simulink model "ResidentialBuildingTESandPVcell"  (R2023b)
settings: Solver=VariableStepAuto  StartTime=0.0  StopTime=3600*24  FixedStep=20  RelTol=1e-3  AbsTol=1e-3
PreLoadFcn:
  | setSystemParams
undefined symbols (not defined in the file): env, hours, htCondDuct, pumps, PVpanel, resUnitParams, tank, wCondDuct
libraries: fl_lib x137, nesl_utility x18, SimscapeFluids_lib x7, simulink x2, ee_lib x2, slpidlib x1
(part 1 of 3)
CloseFcn:
  | clear logsout_ResidentialBuildingTESandPVcell
  | 
  | clear PVpanel heatEx tank pumps TES env resUnitParams simTinit
Description:
  | PV charged sand battery for residential heating
settings Model: Creator=The MathWorks, Inc.  LastModifiedBy=shachind
settings SolverCC: AutoScaleAbsTol=off  MaxConsecutiveMinStep=5  ZeroCrossAlgorithm=Adaptive  AlgebraicLoopSolver=TrustRegion  MaxZcPerStep=1
settings DataIOCC: MaxDataPoints=10000  SaveOutput=off  DSMLogging=off  SaveTime=off  ReturnWorkspaceOutputs=off  SignalLoggingName=logsout_ResidentialBuildingTESandPVcell
settings OptimizationCC: ReuseModelBlockBuffer=off
settings DebuggingCC: ReadBeforeWriteMsg=DisableAll  WriteAfterWriteMsg=DisableAll  WriteAfterReadMsg=DisableAll  IgnoredZcDiagnostic=none  MultiTaskDSMMsg=none  UnconnectedInputMsg=warning  UnconnectedOutputMsg=warning  UnconnectedLineMsg=warning  ArithmeticOperatorsInVariantConditions=warning
settings ModelReferenceCC: UpdateModelReferenceTargets=IfOutOfDate  EnableRefExpFcnMdlSchedulingChecks=on
settings SFSimCC: SFSimEcho=off
settings RTWCC: DLArmComputeVersion=19.05
settings SimscapeCC: SimscapeLogType=all  SimscapeLogSimulationStatistics=on  SimscapeLogName=simlogResidentialBuildingTESandPVcell  SimscapeLogDecimation=10  SimscapeLogLimitData=off  SimscapeLogDataHistory=130000

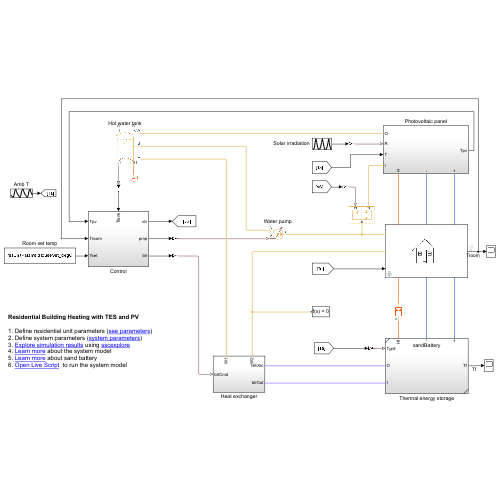
[thumbnail: Simulink's stored preview of the top-level diagram]
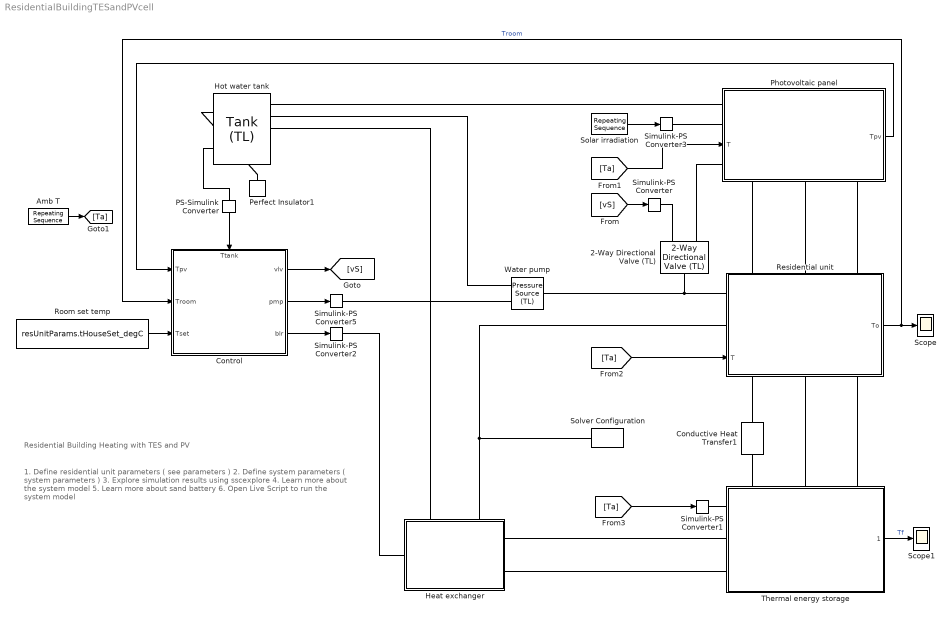
== system ResidentialBuildingTESandPVcell ==
  note: Residential Building Heating with TES and PV
  note: 1. Define residential unit parameters ( see parameters )
      | 2. Define system parameters ( system parameters )
      | 3. Explore simulation results using sscexplore
      | 4. Learn more about the system model
      | 5. Learn more about sand battery
      | 6. Open Live Script to run the system model
  " Water pump" : fl_lib/Thermal Liquid/Sources/Pressure Source (TL)  source_type=foundation.enum.constant_controlled.controlled  pressure_differential=0 MPa  power_spec=foundation.enum.power_spec.isentropic  area=0.01 m^2
      settings: InternalSimscapePortConfiguration="{\"Bottom\":[],\"Left\":[{\"id\":\"A\",\"label\":\"A\",\"type\":\"foundation.thermal_liquid.thermal_liquid\"},{\"id\":\"P\",\"label\":\"P\",\"type\":\"input\"}],\"Right\":[{\"id\":\"B\",\"label\":\"B\",\"type\":\"foundation.thermal_liquid.thermal_liquid\"}],\"Top\":[]}"
  2-Way Directional Valve (TL) : SimscapeFluids_lib/Thermal Liquid/Valves & Orifices/Directional Control Valves/2-Way Directional Valve (TL)  valve_spec=fluids.thermal_liquid.valves.directional_control_valves.enum.ValveSpec.Linear  S_max=5e-2 m  del_S_max=1e-1 m  area_max=2.5e-4 m^2  area_leak=1e-5 m^2  del_S_TLU=[0, .002, .004, .007, .017] m  valve_area_TLU=[1e-09, 2.0352e-07, 4.0736e-05, .00011438, .00034356] m^2  del_S_flow_TLU=[0, .002, .004, .007, .017] m  p_diff_TLU=[.3, .5, .7] MPa  vol_flow_TLU=1e-3 * [1.7e-05, 2e-05, 2.6e-05; .0035, .0045, .0053; .7, .9, 1.06; 1.96, 2.5, 3; 6, 7.7, 9.13] m^3/s  mdot_TLU=[1.7e-05, 2e-05, 2.6e-05; .0035, .0045, .0053; .7, .9, 1.06; 1.96, 2.5, 3; 6, 7.7, 9.13] kg/s  T_ref_in=293.15 K  p_ref_in=0.101325 MPa  Cd=0.7  Re_c=12  smoothing_factor=0.02  pressure_recovery=simscape.enum.onoff.off  area=0.01 m^2
      settings: InternalSimscapePortConfiguration="{\"Bottom\":[],\"Left\":[{\"id\":\"A\",\"label\":\"A\",\"type\":\"foundation.thermal_liquid.thermal_liquid\"}],\"Right\":[{\"id\":\"S\",\"label\":\"S\",\"type\":\"input\"},{\"id\":\"B\",\"label\":\"B\",\"type\":\"foundation.thermal_liquid.thermal_liquid\"}],\"Top\":[]}"
  Amb T : simulink/Sources/Repeating Sequence  rep_seq_t=3600*hours(env.hrs)  rep_seq_y=env.Temp_degC
  Conductive Heat Transfer1 : fl_lib/Thermal/Thermal Elements/Conductive Heat Transfer  thermal_type=foundation.enum.ConstantVariableTabulated.Constant  wall_geometry=foundation.enum.ConductionWallGeometry.Planar  area=TES.pitA m^2  thickness=0.5 m  d_in=0.05 m  d_out=0.1 m  L=1 m  th_cond_min=10 W/(K*m)  th_cond=3.5 W/(K*m)  th_cond_TLU=[413, 401, 392, 383, 371, 357, 342] W/(K*m)  temp_TLU=[200, 273, 400, 600, 800, 1000, 1200] K  T_specify=off  T_priority=None  T=0 K  T_nominal_specify=off  T_nominal_unit=K  T_nominal_value=1  Q_specify=off  Q_priority=None  Q=0 W  Q_nominal_specify=off  Q_nominal_unit=W  Q_nominal_value=1
  Control : Subsystem
      settings: PortSchema="{\"entries\":[{\"content\":{\"sides\":[{\"content\":{\"connectorIds\":[\"In1\",\"In2\",\"In3\"]},\"type\":\"ConnectorPlacement.EquallySpacedRectSide\",\"uuid\":\"94b2e64d-5198-497a-a3ac-7835c1f17d91\"},{\"content\":{\"connectorIds\":[\"Out1\",\"Out2\",\"Out3\"],\"side\":\"RIGHT\"},\"type\":\"ConnectorPlacement.EquallySpacedRectSide\",\"uuid\":\"aae50087-a35d-4e17-a15b-734053a702a5\"},{\"content\":{\"connectorIds\":[\"In4\"],\"side\":\"TOP\"},\"type\":\"ConnectorPlacement.EquallySpacedRectSide\",\"uuid\":\"cdfabfa3-3647-473e-9efb-0f4c40dd4bf4\"}]},\"type\":\"ConnectorPlacement.EquallySpacedConnector\",\"uuid\":\"f6b74bbd-681f-4865-9cfd-f9bd6391df02\"}],\"packageUris\":[\"http://schema.mathworks.com/mf0/Connector/R2020b\"],\"version\":\"1.0\"}"
  Heat exchanger : Subsystem
      settings: PortSchema="{\"entries\":[{\"content\":{\"sides\":[{\"content\":{\"connectorIds\":[\"LConn1\"]},\"type\":\"ConnectorPlacement.EquallySpacedRectSide\",\"uuid\":\"01ab44eb-c12d-4ed2-868c-d9720820a3c1\"},{\"content\":{\"connectorIds\":[\"RConn1\",\"RConn2\"],\"side\":\"RIGHT\"},\"type\":\"ConnectorPlacement.EquallySpacedRectSide\",\"uuid\":\"0fee6253-0b63-4bf2-bc48-ef503382f712\"},{\"content\":{\"connectorIds\":[\"LConn2\",\"LConn3\"],\"side\":\"TOP\"},\"type\":\"ConnectorPlacement.EquallySpacedRectSide\",\"uuid\":\"0da63f1e-723a-4e43-a092-4a52b54a8044\"}]},\"type\":\"ConnectorPlacement.EquallySpacedConnector\",\"uuid\":\"e3ac5915-ab05-4a21-88c5-2d792696c933\"}],\"packageUris\":[\"http://schema.mathworks.com/mf0/Connector/R2020b\"],\"version\":\"1.0\"}"
  Hot water tank : SimscapeFluids_lib/Thermal Liquid/Tanks & Accumulators/Tank (TL)  num_inlet=fluids.thermal_liquid.tanks_accumulators.enum.NumInlet.Three  pressure_spec=foundation.enum.pressure_spec.atmospheric  tank_pressure=0.101325 MPa  volume_spec=fluids.thermal_liquid.tanks_accumulators.enum.TankVolumeSpec.Constant  tank_area=tank.Atank m^2  level_TLU=[0, 3, 5] m  volume_TLU=[0, 4, 6] m^3  inlet_height_A=0.1 m  inlet_area_A=0.01 m^2  inlet_heights_AB=[.1, .01] m  inlet_areas_AB=[.01, .01] m^2  inlet_heights_ABC=[0.6 0.1 0.1] m  inlet_areas_ABC=tank.inAreaVec m^2  inlet_heights_ABCD=[0.75,0.75,0.1,0.1] m  inlet_areas_ABCD=wCondDuct * htCondDuct * ones(1, 4) m^2  inlet_heights_ABCDE=0.1 * ones(1, 5) m  inlet_areas_ABCDE=0.01 * ones(1, 5) m^2  inlet_heights_ABCDEF=0.1 * ones(1, 6) m  inlet_areas_ABCDEF=0.01 * ones(1, 6) m^2  level_check=simscape.enum.assert.action.error  capacity_check=simscape.enum.assert.action.none  max_capacity=tank.Volmax m^3  g=9.81 m/s^2  level_specify=on  level_priority=High  level=tank.Htank0 m  level_nominal_specify=on  level_nominal_unit=m  level_nominal_value=1  volume_specify=off  volume_priority=Low  volume=0.5 m^3  volume_nominal_specify=off  volume_nominal_unit=m^3  volume_nominal_value=1  mass_specify=off  mass_priority=None  mass=5000 kg  mass_nominal_specify=off  mass_nominal_unit=kg  mass_nominal_value=1  T_I_specify=on  T_I_priority=High  T_I=simTinit K  T_I_nominal_specify=on  T_I_nominal_unit=K  T_I_nominal_value=heatEx.water.initTemp
      settings: InternalSimscapePortConfiguration="{\"Bottom\":[{\"id\":\"H\",\"label\":\"H\",\"type\":\"foundation.thermal.thermal\"},{\"id\":\"T_out\",\"label\":\"T\",\"type\":\"output\"}],\"Left\":[{\"id\":\"A\",\"label\":\"A\",\"type\":\"foundation.thermal_liquid.thermal_liquid\"},{\"id\":\"B\",\"label\":\"B\",\"type\":\"foundation.thermal_liquid.thermal_liquid\"},{\"id\":\"C\",\"label\":\"C\",\"type\":\"foundation.thermal_liquid.thermal_liquid\"}],\"Right\":[],\"Top\":[{\"id\":\"V_out\",\"label\":\"V\",\"type\":\"output\"},{\"id\":\"L_out\",\"label\":\"L\",\"type\":\"output\"}]}"
  PS-Simulink Converter : nesl_utility/PS-Simulink Converter  PhysicalDomain=network_engine_domain  SubClassName=ps_output  LeftPortType=input  RightPortType=output  PseudoPeriodic=off  Frequencies=[]  VectorFormat=inherit  Unit=degC  AffineConversion=on
  Perfect Insulator1 : fl_lib/Thermal/Thermal Elements/Perfect Insulator  T_specify=off  T_priority=None  T=80 degC  T_nominal_specify=off  T_nominal_unit=K  T_nominal_value=1
  Photovoltaic panel : Subsystem
      settings: PortSchema="{\"entries\":[{\"content\":{\"sides\":[{\"content\":{\"connectorIds\":[\"LConn1\",\"LConn2\",\"In1\",\"LConn3\"]},\"type\":\"ConnectorPlacement.EquallySpacedRectSide\",\"uuid\":\"0360564f-72df-484c-9030-dc8e52eec76f\"},{\"content\":{\"connectorIds\":[\"Out1\"],\"side\":\"RIGHT\"},\"type\":\"ConnectorPlacement.EquallySpacedRectSide\",\"uuid\":\"6991191b-726f-47c1-9876-cb30d7467486\"},{\"content\":{\"connectorIds\":[],\"side\":\"TOP\"},\"type\":\"ConnectorPlacement.EquallySpacedRectSide\",\"uuid\":\"ebbf2773-9d89-4e6b-a32d-8a074c897184\"},{\"content\":{\"connectorIds\":[\"RConn1\",\"RConn2\",\"RConn3\"],\"side\":\"BOTTOM\"},\"type\":\"ConnectorPlacement.EquallySpacedRectSide\",\"uuid\":\"7a9e78fa-a5b3-4167-9d7a-fcae3edca6f1\"}]},\"type\":\"ConnectorPlacement.EquallySpacedConnector\",\"uuid\":\"26d45dd1-c31c-4c48-b41b-07403e4fd5a3\"}],\"packageUris\":[\"http://schema.mathworks.com/mf0/Connector/R2020b\"],\"version\":\"1.0\"}"
  Residential unit : Subsystem  mask{loadR=9.6941}
      mask prompts: loadR "House Load Resistance"
      settings: PortSchema="{\"entries\":[{\"content\":{\"sides\":[{\"content\":{\"connectorIds\":[\"LConn1\",\"LConn2\",\"In1\"]},\"type\":\"ConnectorPlacement.EquallySpacedRectSide\",\"uuid\":\"97b2c06a-15b0-40ca-95d1-a820c5c9ffc3\"},{\"content\":{\"connectorIds\":[\"Out1\"],\"side\":\"RIGHT\"},\"type\":\"ConnectorPlacement.EquallySpacedRectSide\",\"uuid\":\"71c90047-40c7-4d7b-b242-4c5375799af9\"},{\"content\":{\"connectorIds\":[\"LConn3\",\"LConn4\",\"LConn5\"],\"side\":\"TOP\"},\"type\":\"ConnectorPlacement.EquallySpacedRectSide\",\"uuid\":\"150c8130-4487-4a80-a6e0-fefdc2adbdb9\"},{\"content\":{\"connectorIds\":[\"RConn1\",\"RConn2\",\"RConn3\"],\"side\":\"BOTTOM\"},\"type\":\"ConnectorPlacement.EquallySpacedRectSide\",\"uuid\":\"51ddefcb-2487-47a1-a055-ea39111cb06f\"}]},\"type\":\"ConnectorPlacement.EquallySpacedConnector\",\"uuid\":\"e9cbc702-75ac-4da0-8746-216376f9d2cc\"}],\"packageUris\":[\"http://schema.mathworks.com/mf0/Connector/R2020b\"],\"version\":\"1.0\"}"
  Room set temp : Constant  Value=resUnitParams.tHouseSet_degC
  Scope : Scope
  Scope1 : Scope
  Simulink-PS Converter{,2..3,5} (4 alike) : nesl_utility/Simulink-PS Converter  PhysicalDomain=network_engine_domain  SubClassName=ps_input  LeftPortType=input  RightPortType=output  PseudoPeriodic=off  Frequencies=[]  NoiseDistribution=none  NoiseParameters=[]  Unit=1  AffineConversion=off  FilteringAndDerivatives=provide  SimscapeFilterOrder=1  InputFilterTimeConstant=0.001  UdotUserProvided=0
  Simulink-PS Converter1 : nesl_utility/Simulink-PS Converter  PhysicalDomain=network_engine_domain  SubClassName=ps_input  LeftPortType=input  RightPortType=output  PseudoPeriodic=off  Frequencies=[]  NoiseDistribution=none  NoiseParameters=[]  Unit=degC  AffineConversion=on  FilteringAndDerivatives=filter  SimscapeFilterOrder=1  InputFilterTimeConstant=96  UdotUserProvided=0
  Solar irradiation : simulink/Sources/Repeating Sequence  rep_seq_t=3600*hours(env.hrs)  rep_seq_y=env.slIrr
  Solver Configuration : nesl_utility/Solver Configuration  PhysicalDomain=network_engine_domain  SubClassName=solver  LeftPortType=input  RightPortType=generic  Tones=[]  Harmonics=[]  SimulateNoise=off  Profile=off  UseLocalSampling=off  EnableSwitchedLinearOptims=on  FrequencyDomain=off  UseCCode=off  RelTol=0.001  AbsTol=1e-06  MinStep=1e-09  ToWorkspace=off  RevertToSquareIcSolve=off  NumHomotopyIterations=100  PhasorMode=off  PhasorModeNumHarmonics=1  ConsistencySolver=NEWTON_XTOL_AFTER_FTOL  IndexReductionMethod=DerivativeReplacement  DoDC=off  ResidualTolerance=1e-09  ConsistencyTolSource=GLOBAL  ConsistencyAbsTol=0.001  ConsistencyRelTol=0.001  ConsistencyTolFactor=0.001  UseLocalSolver=off  LocalSolverChoice=NE_BACKWARD_EULER_ADVANCER  ResolveIndetEquations=on  FunctionEvalNumThread=1  LocalSolverSampleTime=60  DoFixedCost=off  MaxNonlinIter=3  MaxModeIter=2  ComputeImpulses=off  ImpulseIterations=2  LinearAlgebra=auto  LinearAlgebraNumThread=0  EquationFormulation=NE_TIME_EF  DelaysMemoryBudget=1024  AutomaticFiltering=on  FilteringTimeConstant=0.001  PartitionStorageMethod=AS_NEEDED  PartitionMemoryBudget=1024  PartitionMethod=ROBUST  MultibodyUseLocalSolver=off  MultibodyLocalSolverChoice=ODE1  MultibodyLocalSolverSampleTime=0.001
  Thermal energy storage : Subsystem  ReferencedSubsystem=sandBattery
      settings: PortSchema="{\"entries\":[{\"content\":{\"sides\":[{\"content\":{\"connectorIds\":[\"LConn1\",\"LConn2\",\"LConn3\"]},\"type\":\"ConnectorPlacement.EquallySpacedRectSide\",\"uuid\":\"edf3f4f8-c2ae-4814-b0e6-abb27056bfc2\"},{\"content\":{\"connectorIds\":[\"Out1\"],\"side\":\"RIGHT\"},\"type\":\"ConnectorPlacement.EquallySpacedRectSide\",\"uuid\":\"77563953-da57-47d3-a930-11c57840b2f6\"},{\"content\":{\"connectorIds\":[\"LConn4\",\"LConn5\",\"LConn6\"],\"side\":\"TOP\"},\"type\":\"ConnectorPlacement.EquallySpacedRectSide\",\"uuid\":\"b81e6b21-ce21-47f9-be2a-ef78bc306350\"},{\"content\":{\"side\":\"BOTTOM\"},\"type\":\"ConnectorPlacement.EquallySpacedRectSide\",\"uuid\":\"24bb3e3d-daaf-432b-aefe-6de5ae56d496\"}]},\"type\":\"ConnectorPlacement.EquallySpacedConnector\",\"uuid\":\"84e32128-2367-4d2f-9f94-d275aa5aafb4\"}],\"packageUris\":[\"http://schema.mathworks.com/mf0/Connector/R2020b\"],\"version\":\"1.0\"}"
  wires:
  Photovoltaic panel/1(Tpv) -> Control/1(Tpv)
  Solar irradiation/1 -> Simulink-PS Converter3/1
  Room set temp/1 -> Control/3(Tset)
  Control/3(blr) -> Simulink-PS Converter2/1
  Control/2(pmp) -> Simulink-PS Converter5/1
  Control/1(vlv) -> [vS]
  [vS] -> Simulink-PS Converter/1
  [Ta] -> Photovoltaic panel/1(T)
  Amb T/1 -> [Ta]
  Residential unit/1(To) -> Control/2(Troom), Scope/1  "Troom"
  [Ta] -> Residential unit/1(T)
  [Ta] -> Simulink-PS Converter1/1
  Thermal energy storage/1 -> Scope1/1  "Tf"
  PS-Simulink Converter/1 -> Control/4(Ttank)
  connections:
  Conductive Heat Transfer1/LConn1 -- Thermal energy storage/LConn4
  Residential unit/LConn3 -- Photovoltaic panel/RConn1
  Simulink-PS Converter3/RConn1 -- Photovoltaic panel/LConn2
  " Water pump"/LConn2 -- Simulink-PS Converter5/RConn1
  Hot water tank/RConn1 -- Perfect Insulator1/LConn1
  Simulink-PS Converter1/RConn1 -- Thermal energy storage/LConn1
  " Water pump"/RConn1 -- Residential unit/LConn1 -- 2-Way Directional Valve (TL)/LConn1
  Simulink-PS Converter/RConn1 -- 2-Way Directional Valve (TL)/RConn1
  Hot water tank/LConn2 -- " Water pump"/LConn1
  Hot water tank/LConn1 -- Photovoltaic panel/LConn1
  2-Way Directional Valve (TL)/RConn2 -- Photovoltaic panel/LConn3
  Residential unit/RConn2 -- Thermal energy storage/LConn5
  Residential unit/RConn3 -- Thermal energy storage/LConn6
  Residential unit/LConn4 -- Photovoltaic panel/RConn2
  Residential unit/LConn5 -- Photovoltaic panel/RConn3
  Residential unit/RConn1 -- Conductive Heat Transfer1/RConn1
  Heat exchanger/LConn2 -- Hot water tank/LConn3
  Solver Configuration/RConn1 -- Residential unit/LConn2 -- Heat exchanger/LConn3
  Heat exchanger/LConn1 -- Simulink-PS Converter2/RConn1
  Heat exchanger/RConn1 -- Thermal energy storage/LConn2
  Heat exchanger/RConn2 -- Thermal energy storage/LConn3
  PS-Simulink Converter/LConn1 -- Hot water tank/RConn2

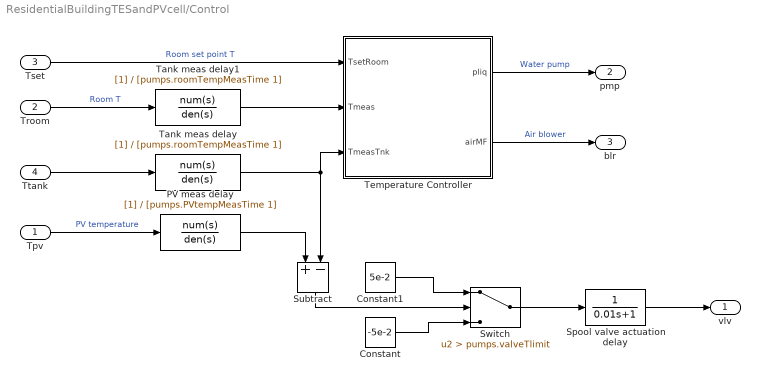
== system ResidentialBuildingTESandPVcell/Control ==
  Tpv : Inport
  Troom : Inport  Port=2
  Tset : Inport  Port=3
  Ttank : Inport  Port=4
  " PV meas delay " : TransferFcn  Denominator=[pumps.PVtempMeasTime 1]
  Constant : Constant  Value=-5e-2
  Constant1 : Constant  Value=5e-2
  "Spool valve actuation delay " : TransferFcn  Denominator=[0.01 1]
  Subtract : Sum  Inputs=+-
  Switch : Switch  Criteria=u2 > Threshold  Threshold=pumps.valveTlimit  ZeroCross=off  SaturateOnIntegerOverflow=off  InputSameDT=off
  Tank meas delay : TransferFcn  Denominator=[pumps.roomTempMeasTime 1]
  Tank meas delay1 : TransferFcn  Denominator=[pumps.roomTempMeasTime 1]
  Temperature Controller : Subsystem
  vlv : Outport
  pmp : Outport  Port=2
  blr : Outport  Port=3
  wires:
  Switch/1 -> "Spool valve actuation delay "/1
  Temperature Controller/2(airMF) -> blr/1  "Air blower"
  " PV meas delay "/1 -> Subtract/1
  Tpv/1 -> " PV meas delay "/1  "PV temperature"
  Constant/1 -> Switch/3
  Subtract/1 -> Switch/2
  Troom/1 -> Tank meas delay1/1  "Room T"
  Constant1/1 -> Switch/1
  Temperature Controller/1(pliq) -> pmp/1  "Water pump"
  "Spool valve actuation delay "/1 -> vlv/1
  Ttank/1 -> Tank meas delay/1
  Tank meas delay/1 -> Temperature Controller/3(TmeasTnk), Subtract/2
  Tset/1 -> Temperature Controller/1(TsetRoom)  "Room set point T"
  Tank meas delay1/1 -> Temperature Controller/2(Tmeas)

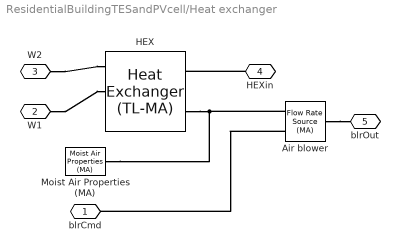
== system ResidentialBuildingTESandPVcell/Heat exchanger ==
  Air blower : fl_lib/Moist Air/Sources/Flow Rate Source (MA)  source_type=foundation.enum.constant_controlled.controlled  flow_type=foundation.enum.mass_volumetric_flow.mass  mass_flow=0 kg/s  volumetric_flow=0 m^3/s  volumetric_flow_conditions=foundation.enum.volumetric_flow_conditions.actual  p_std=0.101325 MPa  T_std=20 degC  RH_std=0.65  power_spec=foundation.enum.power_spec.isentropic  area_A=0.01 m^2  area_B=0.01 m^2
      settings: InternalSimscapePortConfiguration="{\"Bottom\":[],\"Left\":[{\"id\":\"A\",\"label\":\"A\",\"type\":\"foundation.moist_air.moist_air\"},{\"id\":\"M\",\"label\":\"M\",\"type\":\"input\"}],\"Right\":[{\"id\":\"B\",\"label\":\"B\",\"type\":\"foundation.moist_air.moist_air\"}],\"Top\":[]}"
  HEX : SimscapeFluids_lib/Fluid Network Interfaces/Heat Exchangers/Heat Exchanger (TL-MA)  flow_arrangement=fluids.interfaces.heat_exchangers.enum.FlowArrangementTLMA.Cross  cross_flow_arrangement=fluids.interfaces.heat_exchangers.enum.CrossFlowArrangementTLMA.UnmixedMixed  R_wall=0 K/kW  area_A1=heatEx.config.waterInOut m^2  area_B1=heatEx.config.waterInOut m^2  area_A2=heatEx.config.airInOut m^2  area_B2=heatEx.config.airInOut m^2  flow_geometry_TL=fluids.interfaces.heat_exchangers.enum.FlowGeometryTL.InsideTubes  tube_num_TL=heatEx.water.numTube  tube_length_TL=heatEx.water.lenTube m  tube_cross_section_TL=fluids.interfaces.heat_exchangers.enum.TubeCrossSection.Circular  tube_diameter_TL=heatEx.water.diaTube m  tube_width_TL=0.05 m  tube_height_TL=0.05 m  tube_inner_diameter_TL=0.05 m  tube_outer_diameter_TL=0.1 m  tube_flow_area_TL=0.002 m^2  tube_wetted_perimeter_TL=0.15 m  tube_heat_perimeter_TL=0.15 m  tube_pressure_loss_spec_TL=fluids.interfaces.heat_exchangers.enum.TubePressureLossSpec.Haaland  tube_loss_coeff_TL=10  tube_local_pressure_loss_spec_TL=fluids.thermal_liquid.pipes_fittings.enum.LocalLossSpec.AggregateLength  tube_length_add_TL=0.1 m  tube_local_loss_coefficient_TL=0.1  tube_roughness_pressure_TL=15e-6 m  tube_Re_lam_pressure_TL=2000  tube_Re_tur_pressure_TL=4000  tube_shape_factor_generic_TL=64  tube_heat_coeff_spec_TL=fluids.interfaces.heat_exchangers.enum.TubeHeatCoeffSpec.Gneilinski  tube_colburn_coeff_TL=[.023, .8, .33]  tube_roughness_heat_TL=15e-6 m  tube_Re_lam_heat_TL=2000  tube_Re_tur_heat_TL=4000  tube_Nu_lam_generic_TL=3.66  bank_arrangement_TL=fluids.interfaces.heat_exchangers.enum.BankArrangement.Inline  bank_num_rows_TL=5  bank_tubes_per_row_TL=5  bank_width_TL=1 m  bank_tube_diameter_TL=0.05 m  bank_longitudinal_pitch_TL=0.15 m  bank_transverse_pitch_TL=0.15 m  bank_pressure_loss_spec_TL=fluids.interfaces.heat_exchangers.enum.BankPressureLossSpec.Martin  bank_euler_TL=10  bank_heat_coeff_spec_TL=fluids.interfaces.heat_exchangers.enum.BankHeatCoeffSpec.Martin  bank_colburn_coeff_TL=[.27, .63, .36]  generic_flow_area_TL=0.01 m^2  generic_heat_area_TL=2 m^2  generic_volume_TL=0.05 m^3  generic_loss_coeff_TL=10  generic_colburn_coeff_TL=[.023, .8, .33]  fouling_factor_TL=heatEx.water.foulFac K*m^2/kW  fin_area_TL=0 m^2  fin_efficiency_TL=0  p_init_TL=0.109173 MPa  T_init_TL=heatEx.water.initTemp K  flow_geometry_MA=fluids.interfaces.heat_exchangers.enum.FlowGeometryMA.Generic  tube_num_MA=25  tube_length_MA=1 m  tube_cross_section_MA=fluids.interfaces.heat_exchangers.enum.TubeCrossSection.Circular  tube_diameter_MA=0.05 m  tube_width_MA=0.05 m  tube_height_MA=0.05 m  tube_inner_diameter_MA=0.05 m  tube_outer_diameter_MA=0.1 m  tube_flow_area_MA=0.002 m^2  tube_wetted_perimeter_MA=0.15 m  tube_heat_perimeter_MA=0.15 m  tube_pressure_loss_spec_MA=fluids.interfaces.heat_exchangers.enum.TubePressureLossSpec.Haaland  tube_loss_coeff_MA=10  tube_local_pressure_loss_spec_MA=fluids.moist_air.pipes_fittings.enum.LocalLossSpec.AggregateLength  tube_length_add_MA=0.1 m  tube_local_loss_coefficient_MA=0.1  tube_roughness_pressure_MA=15e-6 m  tube_Re_lam_pressure_MA=2000  tube_Re_tur_pressure_MA=4000  tube_shape_factor_generic_MA=64  tube_heat_coeff_spec_MA=fluids.interfaces.heat_exchangers.enum.TubeHeatCoeffSpec.Gneilinski  tube_colburn_coeff_MA=[.023, .8, .33]  tube_roughness_heat_MA=15e-6 m  tube_Re_lam_heat_MA=2000  tube_Re_tur_heat_MA=4000  tube_Nu_lam_generic_MA=3.66  bank_arrangement_MA=fluids.interfaces.heat_exchangers.enum.BankArrangement.Inline  bank_num_rows_MA=15  bank_tubes_per_row_MA=15  bank_width_MA=1 m  bank_tube_diameter_MA=0.05 m  bank_longitudinal_pitch_MA=0.15 m  bank_transverse_pitch_MA=0.15 m  bank_pressure_loss_spec_MA=fluids.interfaces.heat_exchangers.enum.BankPressureLossSpec.Martin  bank_euler_MA=10  bank_heat_coeff_spec_MA=fluids.interfaces.heat_exchangers.enum.BankHeatCoeffSpec.Martin  bank_colburn_coeff_MA=[.27, .63, .36]  generic_flow_area_MA=heatEx.air.minArea m^2  generic_heat_area_MA=heatEx.air.htArea m^2  generic_volume_MA=heatEx.air.volAir m^3  generic_loss_coeff_MA=heatEx.air.prLossC  generic_colburn_coeff_MA=heatEx.air.htcCoff  fouling_factor_MA=0.1 K*m^2/kW  fin_area_MA=heatEx.air.finSur m^2  fin_efficiency_MA=heatEx.air.finEffi  p_init_MA=0.101325 MPa  T_init_MA=heatEx.air.initTemp K  moisture_spec_MA=foundation.enum.moisture_spec.relative_humidity  RH_init_MA=0.5  x_w_init_MA=0.01  y_w_init_MA=0.01  HR_init_MA=0.01  trace_gas_spec_MA=foundation.enum.trace_gas_spec.mass_fraction  x_g_init_MA=0.001  y_g_init_MA=0.001  RH_ws_MA=1
      settings: InternalSimscapePortConfiguration="{\"Bottom\":[],\"Left\":[{\"id\":\"A1\",\"label\":\"A1\",\"type\":\"foundation.thermal_liquid.thermal_liquid\"},{\"id\":\"B1\",\"label\":\"B1\",\"type\":\"foundation.thermal_liquid.thermal_liquid\"}],\"Right\":[{\"id\":\"A2\",\"label\":\"A2\",\"type\":\"foundation.moist_air.moist_air\"},{\"id\":\"B2\",\"label\":\"B2\",\"type\":\"foundation.moist_air.moist_air\"}],\"Top\":[{\"id\":\"W\",\"label\":\"W\",\"type\":\"output\"}]}"
  Moist Air Properties (MA) : fl_lib/Moist Air/Utilities/Moist Air Properties (MA)  R_a=287.047 J/(K*kg)  T_TLU=[-56.55, -50 : 10 : -10, -5 : 1 : 5, 10 : 20 : 700]' degC  h_a_TLU=[342.416126230579; 349.005511058471; 359.063577249119; 369.119948684177; 379.175469465129; 389.230944678417; 394.258910928084; 395.264534937366; 396.27017101329; 397.275819932805; 398.281482472874; 399.287159410541; 400.292851523015; 401.298559587728; 402.304284382408; 403.310026685143; 404.315787274435; 409.34489180313; 419.404921755863; 429.468036401264; 439.535033154839; 449.606720928652; 459.683919949603; 469.767460521911; 479.858181001348; 489.956925196484; 500.064539372946; 510.181869006204; 520.309755403634; 530.449032296018; 540.60052248087; 550.765034584465; 560.943359995745; 571.136270013102; 581.344513234296; 591.568813210327; 601.809866375885; 612.068340261954; 622.344871990218; 632.640067043998; 642.95449830646; 653.288705353699; 663.643193987949; 674.018435994423; 684.414869104228; 694.832897145098; 705.272890361557; 715.735185886199; 726.220088344236; 736.727870574087; 747.258774447567; 757.813011774199] kJ/kg  mu_a_TLU=[14.2568883320012; 14.6140127728333; 15.1517277055779; 15.6806860159119; 16.2012351072083; 16.7137043125028; 16.9670071730589; 17.017438062815; 17.0677930842452; 17.1180725309876; 17.1682766951315; 17.2184058672268; 17.2684603362935; 17.3184403898301; 17.3683463138234; 17.4181783927569; 17.4679369096204; 17.7156358640698; 18.2056751785154; 18.68879035749; 19.1652344664982; 19.6352478927873; 20.099059103658; 20.5568853601578; 21.0089333871663; 21.4554000014051; 21.8964726992323; 22.3323302062775; 22.7631429910631; 23.1890737447833; 23.6102778293792; 24.0269036959922; 24.4390932757886; 24.8469823450548; 25.2507008663546; 25.6503733074314; 26.0461189394339; 26.4380521159325; 26.8262825340948; 27.2109154792923; 27.5920520543128; 27.969789394274; 28.3442208682439; 28.7154362685068; 29.0835219883356; 29.4485611890712; 29.8106339572472; 30.1698174524429; 30.5261860464955; 30.8798114546565; 31.2307628592324; 31.5791070262086] s*uPa  k_a_TLU=[19.8808489374933; 20.4162454629695; 21.2248743590758; 22.0232452890903; 22.8117314495857; 23.5906913619588; 23.9767075412237; 24.053639990175; 24.1304826682191; 24.2072359051629; 24.2839000294007; 24.3604753679152; 24.4369622462801; 24.5133609886625; 24.5896719178249; 24.6658953551279; 24.7420316205333; 25.1214164701832; 25.8738283029331; 26.6180150229276; 27.3542674377332; 28.0828634735341; 28.8040686837224; 29.5181367785657; 30.2253101618423; 30.9258204644224; 31.6198890677835; 32.3077276126633; 32.9895384896798; 33.6655153099498; 34.33584335461; 35.0007000027879; 35.6602551380254; 36.3146715334901; 36.9641052165342; 37.6087058133173; 38.248616874307; 38.8839761815308; 39.5149160384798; 40.1415635435708; 40.7640408480637; 41.3824653993118; 41.9969501701893; 42.6076038755117; 43.2145311762238; 43.8178328720941; 44.4176060836121; 45.013944423749; 45.6069381602018; 46.1966743687041; 46.783237077953; 47.3667074066625] mW/(K*m)  p_min=1 kPa  p_max=inf MPa  T_min=-56.55 degC  T_max=690 degC  properties_range_check=simscape.enum.assert.action.error  p_atm=0.101325 MPa  T_atm=20 degC  R_w=461.523 J/(K*kg)  p_ws_TLU=[1.71168953425982e-06; 3.93770601979424e-06; 1.28411717710344e-05; 3.80051394873809e-05; .00010323902900209; .000259873810798063; .000401741022116384; .000437454836117844; .000476040820618202; .000517704666185737; .000562664883741207; .000611212677444345; .000657088049117899; .000705987905898279; .000758082381149132; .000813549384183233; .000872574861129522; .00122818386934022; .0023392147667769; .00424668834054807; .00738442748706953; .0123512704340234; .0199458019246787; .0312006356960619; .0474147199263783; .0701823607447713; .10141797792131; .143375967241115; .198665399739302; .270259606559999; .361500961984849; .476101381081492; .618139196722055; .792053183687694; 1.0026345688121; 1.25501792086105; 1.55467186826983; 1.90739066433297; 2.31928772772542; 2.79679245576864; 3.34665187151016; 3.97593907083533; 4.69207105435535; 5.5028394740883; 6.41645928168037; 7.4416425436169; 8.58770832955728; 9.86474556030261; 11.2838558865497; 12.8575218898034; 14.6001810568052; 16.5291642526045] MPa  h_w_vap_TLU=[2836.88241275372; 2837.81392500514; 2838.63937175807; 2838.7309929628; 2838.06905313927; 2836.62597341095; 2835.60023952573; 2835.37006381376; 2835.13143158077; 2834.88429145066; 2834.62859062897; 2500.93420564316; 2498.55329907119; 2496.17495082036; 2493.79885912205; 2491.42474723191; 2489.05236104642; 2477.20875029194; 2453.54955988604; 2429.83856603313; 2406.00136954922; 2381.97406342174; 2357.69101156389; 2333.08088387814; 2308.06565480412; 2282.56034405021; 2256.47287422313; 2229.70428017508; 2202.14968030993; 2173.69998896199; 2144.24368406447; 2113.66758247452; 2081.85585110571; 2048.68725710494; 2014.03141249899; 1977.7449923284; 1939.66849592886; 1899.62342931686; 1857.40930169838; 1812.79975416601; 1765.53721731251; 1715.32525772152; 1661.81700477787; 1604.59703745016; 1543.1534616334; 1476.83692476464; 1404.80240352424; 1325.92091736114; 1238.61667822208; 1140.5102987018; 1027.62017777647; 892.733785613825] kJ/kg  h_w_TLU=[2396.55944251649; 2408.68643343608; 2427.1988031141; 2445.702165897; 2464.18429108356; 2482.62529466839; 2491.82135326629; 2493.6580151792; 2495.49372578218; 2497.32843835745; 2499.16210446923; 2500.99462758899; 2502.83092214066; 2504.6665223621; 2506.50140563013; 2508.335548891; 2510.16892865793; 2519.32352241995; 2537.56068088674; 2555.67742615292; 2573.6403223998; 2591.4109179101; 2608.9455037701; 2626.19492016262; 2643.10444358428; 2659.61377634497; 2675.58278696023; 2696.1846256545; 2716.49989553741; 2736.6235210957; 2756.61216047011; 2776.50561773853; 2796.33378922508; 2816.11979583049; 2835.88181423877; 2855.63430574511; 2875.38889327595; 2895.15500577172; 2914.94035964689; 2934.75132290228; 2954.59319330244; 2974.47041285505; 2994.38673458964; 3014.34535328009; 3034.34900867103; 3054.40006755764; 3074.50058946898; 3094.65237953784; 3114.85703128106; 3135.11596137801; 3155.43043805905; 3175.80160435813] kJ/kg  mu_w_TLU=[6.81365662228272; 7.04953750742707; 7.40970098298307; 7.76991278093907; 8.13017290129507; 8.49048134405107; 8.67065368632907; 8.70668960445667; 8.74272600580827; 8.77876289038387; 8.81480025818347; 8.85083810920707; 8.88687644345467; 8.92291526092627; 8.95895456162187; 8.99499434554147; 9.03103461268507; 9.21124319676307; 9.57169660671907; 9.93219833907507; 10.2927483938311; 10.6533467709871; 11.0139934705431; 11.3746884924991; 11.7354318368551; 12.0962235036111; 12.4570634927671; 12.8179518043231; 13.1788884382791; 13.5398733946351; 13.9009066733911; 14.2619882745471; 14.6231181981031; 14.9842964440591; 15.3455230124151; 15.7067979031711; 16.0681211163271; 16.4294926518831; 16.7909125098391; 17.1523806901951; 17.5138971929511; 17.8754620181071; 18.2370751656631; 18.5987366356191; 18.9604464279751; 19.3222045427311; 19.6840109798871; 20.0458657394431; 20.4077688213991; 20.7697202257551; 21.1317199525111; 21.4937680016671] s*uPa  k_w_TLU=[11.46288215976; 11.941997488935; 12.676358586935; 13.414208884935; 14.155548382935; 14.900377080935; 15.274099879935; 15.348949115735; 15.423833243535; 15.498752263335; 15.573706175135; 15.648694978935; 15.723718674735; 15.798777262535; 15.873870742335; 15.948999114135; 16.024162377935; 16.400502076935; 17.155798374935; 17.914583872935; 18.676858570935; 19.442622468935; 20.211875566935; 20.984617864935; 21.760849362935; 22.540570060935; 23.323779958935; 24.110479056935; 24.900667354935; 25.694344852935; 26.491511550935; 27.292167448935; 28.096312546935; 28.903946844935; 29.715070342935; 30.529683040935; 31.347784938935; 32.169376036935; 32.994456334935; 33.823025832935; 34.655084530935; 35.490632428935; 36.329669526935; 37.172195824935; 38.018211322935; 38.867716020935; 39.720709918935; 40.577193016935; 41.437165314935; 42.300626812935; 43.167577510935; 44.038017408935] mW/(K*m)  D_w=25 mm^2/s  trace_gas_model=foundation.enum.trace_gas_model.none  R_g=188.923 J/(K*kg)  h_g_TLU=[439.555216260064; 444.670268200251; 452.538618847003; 460.487124258496; 468.522588768941; 476.649415958793; 480.74798538725; 481.57054318762; 482.394052398751; 483.218514288831; 484.043930029015; 484.870300696555; 485.697627277859; 486.525910671489; 487.355151691079; 488.185351068185; 489.016509455051; 493.186704139431; 501.599194953048; 510.107689961685; 518.711611080182; 527.410026793075; 536.201764778798; 545.085474203452; 554.059675505208; 563.122805485367; 572.27325096919; 581.509373027928; 590.829525105886; 600.232066705818; 609.715373581392; 619.277845178105; 628.917909922924; 638.634028838794; 648.424697859328; 658.288449140109; 668.223851601449; 678.229510889093; 688.304068901113; 698.44620299875; 708.654624994591; 718.928079991818; 729.265345132425; 739.665228299475; 750.126566808087; 760.648226111439; 771.229098541268; 781.868102096908; 792.564179292476; 803.316296068366; 814.123440770426; 824.984623198037] kJ/kg  mu_g_TLU=[10.8921054191698; 11.2215357085649; 11.7233300740382; 12.2234238147811; 12.7215124453467; 13.2173328890673; 13.4643203184773; 13.5136406274989; 13.562934752385; 13.6122025024997; 13.6614436900741; 13.7106581301692; 13.7598456406398; 13.8090060420983; 13.8581391578796; 13.9072448140062; 13.9563228391538; 14.2012926853717; 14.6890687376044; 15.1738428124161; 15.6554929043332; 16.1339159800463; 16.6090257998657; 17.0807510097148; 17.5490334645512; 18.0138267508952; 18.4750948814453; 18.9328111390399; 19.3869570507278; 19.8375214755778; 20.2844997922255; 20.7278931741254; 21.1677079421287; 21.6039549853963; 22.036649242835; 22.4658092382469; 22.8914566632375; 23.3136160026627; 23.7323141980278; 24.1475803447965; 24.5594454200432; 24.9679420372927; 25.3731042257492; 25.774967231431; 26.1735673380029; 26.5689417053362; 26.9611282240413; 27.350165384404; 27.73609215832; 28.118947892972; 28.4987722151178; 28.8756049449796] s*uPa  k_g_TLU=[10.489430678843; 10.9507672150864; 11.666197960308; 12.392559739764; 13.1299519771612; 13.8778409888416; 14.2554325416312; 14.3312274189707; 14.4071122346908; 14.4830860227061; 14.5591478179508; 14.6352966574703; 14.7115315815553; 14.787851634907; 14.8642558678259; 14.9407433374142; 15.0173131087819; 15.401364480906; 16.1751373988038; 16.9558134611595; 17.7432208682398; 18.5366976599676; 19.3360988502003; 20.1412225692689; 20.9517507672929; 21.7672310558863; 22.5871115634685; 23.4107980865695; 24.2377021890869; 25.0672663781241; 25.8989689893876; 26.732318357514; 27.5668446164644; 28.4020933015927; 29.2376215872816; 30.0729965057542; 30.9077942826816; 31.7416001931033; 32.5740086297993; 33.4046232539953; 34.2330571812868; 35.0589331874899; 35.8818839295189; 36.701552179391; 37.5175910702657; 38.3296643536716; 39.1374466671854; 39.9406238119064; 40.7388930391313; 41.5319633456945; 42.3195557774861; 43.1014037407076] mW/(K*m)  D_g=16 mm^2/s
  blrCmd : PMIOPort  Side=Left
  W1 : PMIOPort  Port=2  Side=Left
  W2 : PMIOPort  Port=3  Side=Left
  HEXin : PMIOPort  Port=4  Side=Right
  blrOut : PMIOPort  Port=5  Side=Right
  connections:
  W2/RConn1 -- HEX/LConn1
  HEX/RConn2 -- Air blower/LConn1 -- Moist Air Properties (MA)/RConn1
  Air blower/LConn2 -- blrCmd/RConn1
  Air blower/RConn1 -- blrOut/RConn1
  W1/RConn1 -- HEX/LConn2
  HEXin/RConn1 -- HEX/RConn1

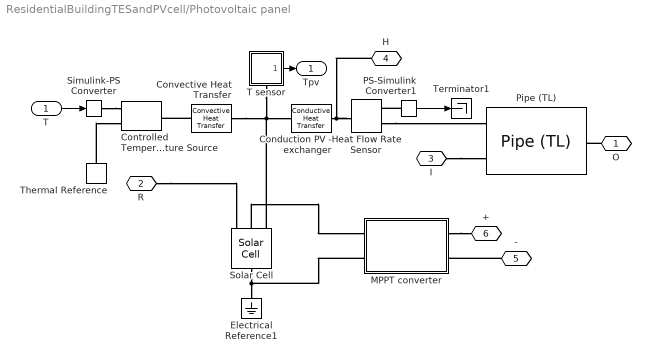
== system ResidentialBuildingTESandPVcell/Photovoltaic panel ==
  T : Inport
  Conduction PV - exchanger : fl_lib/Thermal/Thermal Elements/Conductive Heat Transfer  thermal_type=foundation.enum.ConstantVariableTabulated.Constant  wall_geometry=foundation.enum.ConductionWallGeometry.Planar  area=PVpanel.geometry.areaPanel*PVpanel.geometry.nPrlStr m^2  thickness=PVpanel.heatTransfer.Le m  d_in=0.05 m  d_out=0.1 m  L=1 m  th_cond_min=10 W/(K*m)  th_cond=PVpanel.heatTransfer.ke W/(m*K)  th_cond_TLU=[413, 401, 392, 383, 371, 357, 342] W/(K*m)  temp_TLU=[200, 273, 400, 600, 800, 1000, 1200] K  T_specify=off  T_priority=None  T=0 K  T_nominal_specify=off  T_nominal_unit=K  T_nominal_value=1  Q_specify=off  Q_priority=None  Q=0 W  Q_nominal_specify=off  Q_nominal_unit=W  Q_nominal_value=1
  Controlled Temperature Source : fl_lib/Thermal/Thermal Sources/Controlled Temperature Source
  Convective Heat Transfer : fl_lib/Thermal/Thermal Elements/Convective Heat Transfer  thermal_type=foundation.enum.constant_variable.constant  area=PVpanel.geometry.areaPanel*PVpanel.geometry.nPrlStr m^2  heat_tr_coeff=5 W/(K*m^2)  min_heat_tr_coeff=1e-3 W/(K*m^2)  T_specify=off  T_priority=None  T=0 K  T_nominal_specify=off  T_nominal_unit=K  T_nominal_value=1  Q_specify=off  Q_priority=None  Q=0 W  Q_nominal_specify=off  Q_nominal_unit=W  Q_nominal_value=1
  Electrical Reference1 : fl_lib/Electrical/Electrical Elements/Electrical Reference
  Heat Flow Rate Sensor : fl_lib/Thermal/Thermal Sensors/Heat Flow Rate Sensor
  MPPT converter : Subsystem  mask(Simplified Solar PV Converter){Rload=PVpanel.MPPTRes, Vm=38.8}
      mask prompts: Rload "Load resistance (Ohm)"; Vm "Maximum power point voltage (V)"
  PS-Simulink Converter1 : nesl_utility/PS-Simulink Converter  PhysicalDomain=network_engine_domain  SubClassName=ps_output  LeftPortType=input  RightPortType=output  PseudoPeriodic=off  Frequencies=[]  VectorFormat=inherit  Unit=inherit  AffineConversion=off
  Pipe (TL) : fl_lib/Thermal Liquid/Elements/Pipe (TL)  length=PVpanel.geometry.areaPanel*PVpanel.geometry.nPrlStr/sqrt(PVpanel.heatTransfer.tubeCS) m  area=PVpanel.heatTransfer.tubeCS m^2  Dh=PVpanel.heatTransfer.tubeHD m  length_add=1 m  roughness=15e-6 m  Re_lam=2000  Re_tur=4000  shape_factor=64  Nu_lam=3.66  dynamic_compressibility=simscape.enum.onoff.off  inertia=simscape.enum.onoff.off  p0=0.101325 MPa  T0=simTinit K  mdot0=0 kg/s
  Simulink-PS Converter : nesl_utility/Simulink-PS Converter  PhysicalDomain=network_engine_domain  SubClassName=ps_input  LeftPortType=input  RightPortType=output  PseudoPeriodic=off  Frequencies=[]  NoiseDistribution=none  NoiseParameters=[]  Unit=degC  AffineConversion=on  FilteringAndDerivatives=provide  SimscapeFilterOrder=1  InputFilterTimeConstant=0.001  UdotUserProvided=0
  Solar Cell : ee_lib/Sources/Solar Cell  Tag={'toolbox/physmod/elec/library/m/ee_lib_parts';'Sources/Solar_Cell/Amerisolar/AS_6M_360W_PERC.xml'}  prm=3  Isc=9.64 A  Voc=0.65833 V  Is=3.26005689221038e-07 A  Is2=2.08812935747622e-09 A  Iph=9.64000663446818 A  Ir0=1000 W/m^2  ec=1.48955183509565  N2=2.03537290915688  Rs=0.000587128359683705 Ohm  Rp=771.966793824014 Ohm  N_series=PVpanel.geometry.nSeries  N_parallel=PVpanel.geometry.nPrlStr  TIPH1=0.000519981408860291 1/K  EG=1.12 eV  TXIS1=4.17598231137541  TXIS2=18.4602091098286  TRS1=0.101104089054628  TRP1=0 % Parameter not set  Tmeas=25 degC  TFIXED=25 degC  thermal_mass=100 % Parameter not set J/K  initial_temperature=simTinit K
      settings: AttributesFormatString=Amerisolar:AS_6M_360W_PERC  InternalSimscapePortConfiguration="{\"Bottom\":[],\"Left\":[{\"id\":\"Ir\",\"label\":\"Ir\",\"type\":\"input\"},{\"id\":\"p\",\"label\":\"+\",\"type\":\"foundation.electrical.electrical\"},{\"id\":\"H\",\"label\":\"H\",\"type\":\"foundation.thermal.thermal\"}],\"Right\":[{\"id\":\"n\",\"label\":\"-\",\"type\":\"foundation.electrical.electrical\"}],\"Top\":[]}"
  T sensor : Subsystem
      settings: PortSchema="{\"entries\":[{\"content\":{\"sides\":[{\"content\":{\"connectorIds\":[\"LConn1\"]},\"type\":\"ConnectorPlacement.EquallySpacedRectSide\",\"uuid\":\"68c07b44-9c16-4a15-b6ea-14dc3535499e\"},{\"content\":{\"connectorIds\":[],\"side\":\"RIGHT\"},\"type\":\"ConnectorPlacement.EquallySpacedRectSide\",\"uuid\":\"10b15f80-9f6a-4bc7-a4ae-eef587b351cc\"},{\"content\":{\"connectorIds\":[],\"side\":\"TOP\"},\"type\":\"ConnectorPlacement.EquallySpacedRectSide\",\"uuid\":\"7bbff4e6-8f68-4967-927e-9d5ec988cf6b\"},{\"content\":{\"connectorIds\":[\"Out1\"],\"side\":\"BOTTOM\"},\"type\":\"ConnectorPlacement.EquallySpacedRectSide\",\"uuid\":\"88c3c9ba-d380-4cf6-9bb3-19e6025022d5\"}]},\"type\":\"ConnectorPlacement.EquallySpacedConnector\",\"uuid\":\"af46a50d-e068-47f9-b4a8-f48b93b1cd77\"}],\"packageUris\":[\"http://schema.mathworks.com/mf0/Connector/R2020b\"],\"version\":\"1.0\"}"
  Terminator1 : Terminator
  Thermal Reference : fl_lib/Thermal/Thermal Elements/Thermal Reference
  O : PMIOPort  Side=Left
  R : PMIOPort  Port=2  Side=Left
  I : PMIOPort  Port=3  Side=Left
  H : PMIOPort  Port=4  Side=Right
  - : PMIOPort  Port=5  Side=Right
  + : PMIOPort  Port=6  Side=Right
  Tpv : Outport
  wires:
  T/1 -> Simulink-PS Converter/1
  T sensor/1(Tpv) -> Tpv/1
  PS-Simulink Converter1/1 -> Terminator1/1
  connections:
  Convective Heat Transfer/LConn1 -- Solar Cell/LConn3 -- T sensor/LConn1 -- Conduction PV - exchanger/LConn1
  Conduction PV - exchanger/RConn1 -- H/RConn1 -- Heat Flow Rate Sensor/LConn1
  Solar Cell/RConn1 -- MPPT converter/LConn2 -- Electrical Reference1/LConn1
  R/RConn1 -- Solar Cell/LConn1
  PS-Simulink Converter1/LConn1 -- Heat Flow Rate Sensor/RConn1
  Heat Flow Rate Sensor/RConn2 -- Pipe (TL)/LConn2
  Simulink-PS Converter/RConn1 -- Controlled Temperature Source/RConn1
  Thermal Reference/LConn1 -- Controlled Temperature Source/RConn2
  Convective Heat Transfer/RConn1 -- Controlled Temperature Source/LConn1
  O/RConn1 -- Pipe (TL)/RConn1
  I/RConn1 -- Pipe (TL)/LConn1
  Solar Cell/LConn2 -- MPPT converter/LConn1
  -/RConn1 -- MPPT converter/RConn2
  MPPT converter/RConn1 -- +/RConn1

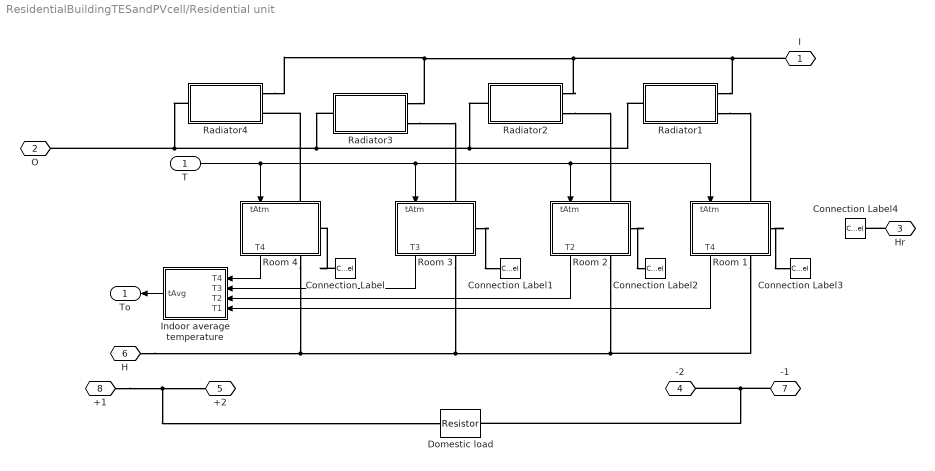
== system ResidentialBuildingTESandPVcell/Residential unit ==
  T : Inport
  Connection Label{,1..4} (5 alike) : ConnectionLabel  Label=Hr1
  Domestic load : fl_lib/Electrical/Electrical Elements/Resistor  R=loadR Ohm  i_specify=off  i_priority=None  i=0 A  i_nominal_specify=off  i_nominal_unit=A  i_nominal_value=1  v_specify=off  v_priority=None  v=0 V  v_nominal_specify=off  v_nominal_unit=V  v_nominal_value=1
  Indoor average temperature : Subsystem
  Radiator1 : Subsystem  mask{pow=resUnitParams.radiator.powerRating, tubeDia=resUnitParams.radiator.diaPipe, htc=resUnitParams.radiator.hRoomAir}
      mask prompts: pow "Power rating (BTU/hr)"; tubeDia "Tube dia(mm)"; htc "Convection HTC (W/K-m^2)"
      mask DialogControl RadiatorParam Prompt: Radiator
  Radiator2 : Subsystem  mask{pow=resUnitParams.radiator.powerRating, tubeDia=resUnitParams.radiator.diaPipe, htc=resUnitParams.radiator.hRoomAir}
      mask prompts: pow "Power rating (BTU/hr)"; tubeDia "Tube dia(mm)"; htc "Convection HTC (W/K-m^2)"
      mask DialogControl RadiatorParam Prompt: Radiator
  Radiator3 : Subsystem  mask{pow=resUnitParams.radiator.powerRating, tubeDia=resUnitParams.radiator.diaPipe, htc=resUnitParams.radiator.hRoomAir}
      mask prompts: pow "Power rating (BTU/hr)"; tubeDia "Tube dia(mm)"; htc "Convection HTC (W/K-m^2)"
      mask DialogControl RadiatorParam Prompt: Radiator
  Radiator4 : Subsystem  mask{pow=resUnitParams.radiator.powerRating, tubeDia=resUnitParams.radiator.diaPipe, htc=resUnitParams.radiator.hRoomAir}
      mask prompts: pow "Power rating (BTU/hr)"; tubeDia "Tube dia(mm)"; htc "Convection HTC (W/K-m^2)"
      mask DialogControl RadiatorParam Prompt: Radiator
  Room 1 : Subsystem  Tag=PublishSubsystem
      settings: PortSchema="{\"entries\":[{\"content\":{\"sides\":[{\"content\":{\"connectorIds\":[\"In1\",\"LConn1\"]},\"type\":\"ConnectorPlacement.EquallySpacedRectSide\",\"uuid\":\"b82312fb-1d28-4e74-b040-1bbc3aeb736a\"},{\"content\":{\"connectorIds\":[\"Out1\",\"RConn1\"],\"side\":\"RIGHT\"},\"type\":\"ConnectorPlacement.EquallySpacedRectSide\",\"uuid\":\"7362106d-0819-49fa-9f99-6c3c7d4a3932\"},{\"content\":{\"connectorIds\":[],\"side\":\"TOP\"},\"type\":\"ConnectorPlacement.EquallySpacedRectSide\",\"uuid\":\"1595a556-c4e6-4bf4-89e6-4336e14d434f\"},{\"content\":{\"connectorIds\":[\"RConn2\"],\"side\":\"BOTTOM\"},\"type\":\"ConnectorPlacement.EquallySpacedRectSide\",\"uuid\":\"afb75a58-dadf-43f1-967c-fbdbdf84975f\"}]},\"type\":\"ConnectorPlacement.EquallySpacedConnector\",\"uuid\":\"09432d56-1749-4d6a-af33-bf3b474a49af\"}],\"packageUris\":[\"http://schema.mathworks.com/mf0/Connector/R2020b\"],\"version\":\"1.0\"}"
  Room 2 : Subsystem  Tag=PublishSubsystem
      settings: PortSchema="{\"entries\":[{\"content\":{\"sides\":[{\"content\":{\"connectorIds\":[\"In1\",\"LConn1\"]},\"type\":\"ConnectorPlacement.EquallySpacedRectSide\",\"uuid\":\"b82312fb-1d28-4e74-b040-1bbc3aeb736a\"},{\"content\":{\"connectorIds\":[\"Out1\",\"RConn1\"],\"side\":\"RIGHT\"},\"type\":\"ConnectorPlacement.EquallySpacedRectSide\",\"uuid\":\"7362106d-0819-49fa-9f99-6c3c7d4a3932\"},{\"content\":{\"connectorIds\":[],\"side\":\"TOP\"},\"type\":\"ConnectorPlacement.EquallySpacedRectSide\",\"uuid\":\"1595a556-c4e6-4bf4-89e6-4336e14d434f\"},{\"content\":{\"connectorIds\":[\"RConn2\"],\"side\":\"BOTTOM\"},\"type\":\"ConnectorPlacement.EquallySpacedRectSide\",\"uuid\":\"afb75a58-dadf-43f1-967c-fbdbdf84975f\"}]},\"type\":\"ConnectorPlacement.EquallySpacedConnector\",\"uuid\":\"09432d56-1749-4d6a-af33-bf3b474a49af\"}],\"packageUris\":[\"http://schema.mathworks.com/mf0/Connector/R2020b\"],\"version\":\"1.0\"}"
  "Room 3 " : Subsystem  Tag=PublishSubsystem
      settings: PortSchema="{\"entries\":[{\"content\":{\"sides\":[{\"content\":{\"connectorIds\":[\"In1\",\"LConn1\"]},\"type\":\"ConnectorPlacement.EquallySpacedRectSide\",\"uuid\":\"b82312fb-1d28-4e74-b040-1bbc3aeb736a\"},{\"content\":{\"connectorIds\":[\"Out1\",\"RConn1\"],\"side\":\"RIGHT\"},\"type\":\"ConnectorPlacement.EquallySpacedRectSide\",\"uuid\":\"7362106d-0819-49fa-9f99-6c3c7d4a3932\"},{\"content\":{\"connectorIds\":[],\"side\":\"TOP\"},\"type\":\"ConnectorPlacement.EquallySpacedRectSide\",\"uuid\":\"1595a556-c4e6-4bf4-89e6-4336e14d434f\"},{\"content\":{\"connectorIds\":[\"RConn2\"],\"side\":\"BOTTOM\"},\"type\":\"ConnectorPlacement.EquallySpacedRectSide\",\"uuid\":\"afb75a58-dadf-43f1-967c-fbdbdf84975f\"}]},\"type\":\"ConnectorPlacement.EquallySpacedConnector\",\"uuid\":\"09432d56-1749-4d6a-af33-bf3b474a49af\"}],\"packageUris\":[\"http://schema.mathworks.com/mf0/Connector/R2020b\"],\"version\":\"1.0\"}"
  Room 4 : Subsystem  Tag=PublishSubsystem
      settings: PortSchema="{\"entries\":[{\"content\":{\"sides\":[{\"content\":{\"connectorIds\":[\"In1\",\"LConn1\"]},\"type\":\"ConnectorPlacement.EquallySpacedRectSide\",\"uuid\":\"b82312fb-1d28-4e74-b040-1bbc3aeb736a\"},{\"content\":{\"connectorIds\":[\"Out1\",\"RConn1\"],\"side\":\"RIGHT\"},\"type\":\"ConnectorPlacement.EquallySpacedRectSide\",\"uuid\":\"7362106d-0819-49fa-9f99-6c3c7d4a3932\"},{\"content\":{\"connectorIds\":[],\"side\":\"TOP\"},\"type\":\"ConnectorPlacement.EquallySpacedRectSide\",\"uuid\":\"1595a556-c4e6-4bf4-89e6-4336e14d434f\"},{\"content\":{\"connectorIds\":[\"RConn2\"],\"side\":\"BOTTOM\"},\"type\":\"ConnectorPlacement.EquallySpacedRectSide\",\"uuid\":\"afb75a58-dadf-43f1-967c-fbdbdf84975f\"}]},\"type\":\"ConnectorPlacement.EquallySpacedConnector\",\"uuid\":\"09432d56-1749-4d6a-af33-bf3b474a49af\"}],\"packageUris\":[\"http://schema.mathworks.com/mf0/Connector/R2020b\"],\"version\":\"1.0\"}"
  I : PMIOPort  Side=Left
  O : PMIOPort  Port=2  Side=Left
  Hr : PMIOPort  Port=3  Side=Left
  -2 : PMIOPort  Port=4  Side=Left
  +2 : PMIOPort  Port=5  Side=Left
  H : PMIOPort  Port=6  Side=Right
  -1 : PMIOPort  Port=7  Side=Right
  +1 : PMIOPort  Port=8  Side=Right
  To : Outport  VectorParamsAs1DForOutWhenUnconnected=off
  wires:
  Room 1/1(T4) -> Indoor average temperature/4(T1)
  "Room 3 "/1(T3) -> Indoor average temperature/2(T3)
  Room 2/1(T2) -> Indoor average temperature/3(T2)
  T/1 -> "Room 3 "/1(tAtm), Room 1/1(tAtm), Room 2/1(tAtm), Room 4/1(tAtm)
  Indoor average temperature/1(tAvg) -> To/1
  Room 4/1(T4) -> Indoor average temperature/1(T4)
  connections:
  Radiator4/LConn1 -- Radiator3/LConn1 -- Radiator2/LConn1 -- Radiator1/LConn1 -- I/RConn1
  Radiator3/RConn1 -- Radiator1/RConn1 -- Radiator2/RConn1 -- Radiator4/RConn1 -- O/RConn1
  Room 4/LConn1 -- Radiator4/LConn2
  Room 4/RConn1 -- H/RConn1 -- Room 1/RConn1 -- Room 2/RConn1 -- "Room 3 "/RConn1
  Connection Label/LConn1 -- Room 4/RConn2
  "Room 3 "/RConn2 -- Connection Label1/LConn1
  Room 2/RConn2 -- Connection Label2/LConn1
  Room 1/RConn2 -- Connection Label3/LConn1
  Hr/RConn1 -- Connection Label4/LConn1
  +1/RConn1 -- Domestic load/LConn1 -- +2/RConn1
  Radiator1/LConn2 -- Room 1/LConn1
  Radiator2/LConn2 -- Room 2/LConn1
  Radiator3/LConn2 -- "Room 3 "/LConn1
  -1/RConn1 -- Domestic load/RConn1 -- -2/RConn1
